simulink model "multiRobotSoccer"  (R2022b)
settings: Solver=FixedStepAuto  StartTime=0.0  StopTime=inf  FixedStep=sampleTime  RelTol=1e-3
PreLoadFcn:
  | robotSoccerParams;
values from neighbouring files (symbols this model uses):
  angThresh = pi/16    (= 0.196349540849)    [robotSoccerParams.m]
  attackerKickSpeed = 3    [robotSoccerParams.m]
  attackerMaxGoalDist = 10    [robotSoccerParams.m]
  attackerMinGoalDist = 5    [robotSoccerParams.m]
  awayGoalPosition = [fieldLimitsX(2) mean(fieldLimitsY)]    [robotSoccerParams.m]
  ballAngleNoise = pi/24    (= 0.1308996939)    [robotSoccerParams.m]
  ballThresh = robotRadius + 0.3    (= 1.1)    [robotSoccerParams.m]
  ballVelNoise = 0.5    [robotSoccerParams.m]
  defenderAwayPoses = [82 28.5 pi ... (first row only)    [robotSoccerParams.m]
  defenderHomePoses = [10 28.5 0 ... (first row only)    [robotSoccerParams.m]
  defenderKickSpeed = 5    [robotSoccerParams.m]
  distThresh = 1    [robotSoccerParams.m]
  dribbleKickSpeed = 2    [robotSoccerParams.m]
  dribbleTime = 25    [robotSoccerParams.m]
  fieldCenter = [mean(fieldLimitsX) mean(fieldLimitsY)]    [robotSoccerParams.m]
  fieldLimitsX = [0 92]    [robotSoccerParams.m]
  fieldLimitsY = [0 47]    [robotSoccerParams.m]
  goalkeeperKickSpeed = 10    [robotSoccerParams.m]
  goalkeeperPoses = [ 2 23.5 0 ... (first row only)    [robotSoccerParams.m]
  goalPosts = [ 0 33 2 ... (first row only)    [robotSoccerParams.m]
  goalThresh = 20    [robotSoccerParams.m]
  homeGoalPosition = [fieldLimitsX(1) mean(fieldLimitsY)]    [robotSoccerParams.m]
  initBallPos = fieldCenter    [robotSoccerParams.m]
  initGameState = struct('possession',0,                         'state',GameState.InPlay,                         'score',[0;0])    [robotSoccerParams.m]
  numRobots = 8    [robotSoccerParams.m]
  objColors = [0 0.75 0; 1 0 0; 0 0 1]    [robotSoccerParams.m]
  objMarkers = 'o^^'    [robotSoccerParams.m]
  outOfBoundsDist = 2    [robotSoccerParams.m]
  robotDetectorMaxHits = 5    [robotSoccerParams.m]
  robotRadius = 0.8    [robotSoccerParams.m]
undefined symbols (not defined in the file or in its folder): DiscIntNeverNeededParam, ObjectType
libraries: soccerRobotLib x8
(part 1 of 2)
settings Model: PacingRate=3  TunableVars=angThresh,attackerKickSpeed,attackerMaxGoalDist,attackerMinGoalDist,awayGoalPosition,ballAngleNoise,ballCarryFactor,ballThresh,ballVelNoise,defenderAwayPoses,defenderHomePoses,defenderKickSpeed,distThresh,dribbleKickSpeed,dribbleTime,fieldCenter,fieldLimitsX,fieldLimitsY,goalPosts,goalThresh,goalkeeperKickSpeed,goalkeeperPoses,homeGoalPosition,initBallPos,initGameState,initialPoses,numRobots,objColors,objDetectorAngle,objDetectorFOV,objDetectorMaxHits,objDetectorOffset,objDetectorRange,outOfBoundsDist,robotColors,robotDetectorAngle,robotDetectorFOV,robotDetectorMaxHits,robotDetectorOffset,robotDetectorRange,robotRadius,sampleTime,wheelRadius  TunableVarsStorageClass=Auto,Auto,Auto,Auto,Auto,Auto,Auto,Auto,Auto,Auto,Auto,Auto,Auto,Auto,Auto,Auto,Auto,Auto,Auto,Auto,Auto,Auto,Auto,Auto,Auto,Auto,Auto,Auto,Auto,Auto,Auto,Auto,Auto,Auto,Auto,Auto,Auto,Auto,Auto,Auto,Auto,Auto,Auto  TunableVarsTypeQualifier=,,,,,,,,,,,,,,,,,,,,,,,,,,,,,,,,,,,,,,,,,,  Creator=scastro  LastModifiedBy=josep
settings SolverCC: AlgebraicLoopSolver=TrustRegion
settings DataIOCC: ReturnWorkspaceOutputs=off
settings OptimizationCC: EnhancedBackFolding=on  PassReuseOutputArgsAs=Individual arguments  OptimizeBlockOrder=speed  DifferentSizesBufferReuse=on  OptimizationCustomize=off  EfficientTunableParamExpr=on
settings DebuggingCC: ParameterTunabilityLossMsg=error  UnconnectedInputMsg=warning  UnconnectedOutputMsg=warning  UnconnectedLineMsg=warning  BusObjectLabelMismatch=error  StrictBusMsg=ErrorOnBusTreatedAsVector  NonBusSignalsTreatedAsBus=error  SFMachineParentedDataDiag=warning  ArithmeticOperatorsInVariantConditions=warning
settings ModelReferenceCC: EnableRefExpFcnMdlSchedulingChecks=on
settings SFSimCC: SimUseLocalCustomCode=off  MATLABDynamicMemAlloc=off  CustomCodeUndefinedFunction=UseInterfaceOnly
settings RTWCC: Description=Embedded Coder  SystemTargetFile=ert.tlc  TemplateMakefile=ert_default_tmf  GenerateReport=on  RTWUseLocalCustomCode=off  IncludeHyperlinkInReport=on  LaunchReport=on  GenerateTraceInfo=on  GenerateTraceReport=on  GenerateTraceReportSl=on  GenerateTraceReportSf=on  GenerateTraceReportEml=on  GenerateWebview=on
settings CodeAppCC: ForceParamTrailComments=on  IgnoreCustomStorageClasses=off  OperatorAnnotations=on  SimulinkDataObjDesc=on  SFDataObjDesc=on  InsertBlockDesc=on
settings ERTTargetCC: TargetLangStandard=C99 (ISO)  GenerateSampleERTMain=on  SupportVariableSizeSignals=on  ERTCustomFileTemplate=example_file_process.tlc

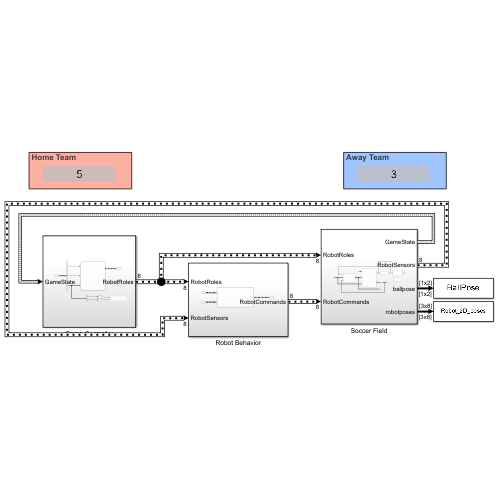
[thumbnail: Simulink's stored preview of the top-level diagram]
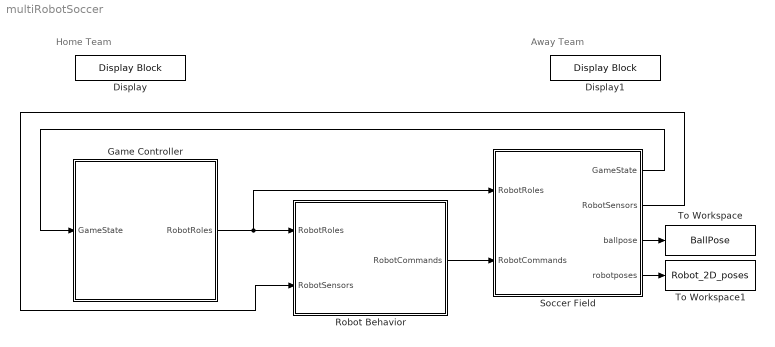
== system multiRobotSoccer ==
  note: Home Team
  note: Away Team
  Display : DisplayBlock  LabelPosition=Hide  Format=long
  Display1 : DisplayBlock  LabelPosition=Hide  Format=long
  Game Controller : Subsystem
  Robot Behavior : Subsystem
  Soccer Field : Subsystem
  To Workspace : ToWorkspace  VariableName=BallPose  SaveFormat=Structure With Time  SampleTime=-1
  To Workspace1 : ToWorkspace  VariableName=Robot_2D_poses  SaveFormat=Structure With Time  SampleTime=-1
  wires:
  Robot Behavior/1(RobotCommands) -> Soccer Field/2(RobotCommands)
  Game Controller/1(RobotRoles) -> Soccer Field/1(RobotRoles), Robot Behavior/1(RobotRoles)
  Soccer Field/1(GameState) -> Game Controller/1(GameState)
  Soccer Field/2(RobotSensors) -> Robot Behavior/2(RobotSensors)
  Soccer Field/3(ballpose) -> To Workspace/1
  Soccer Field/4(robotposes) -> To Workspace1/1

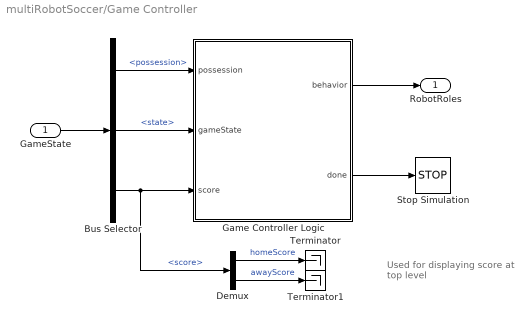
== system multiRobotSoccer/Game Controller ==
  note: Used for displaying score at top level
  GameState : Inport
  Bus Selector : BusSelector  OutputSignals=possession,state,score
  Demux : Demux  Outputs=2
  Game Controller Logic : Stateflow chart  TreatAsAtomicUnit=on
  Stop Simulation : Stop
  Terminator : Terminator
  Terminator1 : Terminator
  RobotRoles : Outport  VectorParamsAs1DForOutWhenUnconnected=off
  wires:
  Game Controller Logic/1(behavior) -> RobotRoles/1
  GameState/1 -> Bus Selector/1
  Bus Selector/1 -> Game Controller Logic/1(possession)  "<possession>"
  Bus Selector/2 -> Game Controller Logic/2(gameState)  "<state>"
  Bus Selector/3 -> Demux/1, Game Controller Logic/3(score)  "<score>"
  Demux/1 -> Terminator/1  "homeScore"
  Demux/2 -> Terminator1/1  "awayScore"
  Game Controller Logic/2(done) -> Stop Simulation/1

== system multiRobotSoccer/Robot Behavior ==
  RobotRoles : Inport
  RobotSensors : Inport  Port=2
  For Each Subsystem (Iterates through all robots) : Subsystem  TreatAsAtomicUnit=on
  RobotCommands : Outport  OutDataTypeStr=Bus: RobotCommandBus  PortDimensions=2  VectorParamsAs1DForOutWhenUnconnected=off
  wires:
  RobotRoles/1 -> For Each Subsystem (Iterates through all robots)/1(robotRoles)
  RobotSensors/1 -> For Each Subsystem (Iterates through all robots)/2(robotSensors)
  For Each Subsystem (Iterates through all robots)/1(robotCommands) -> RobotCommands/1

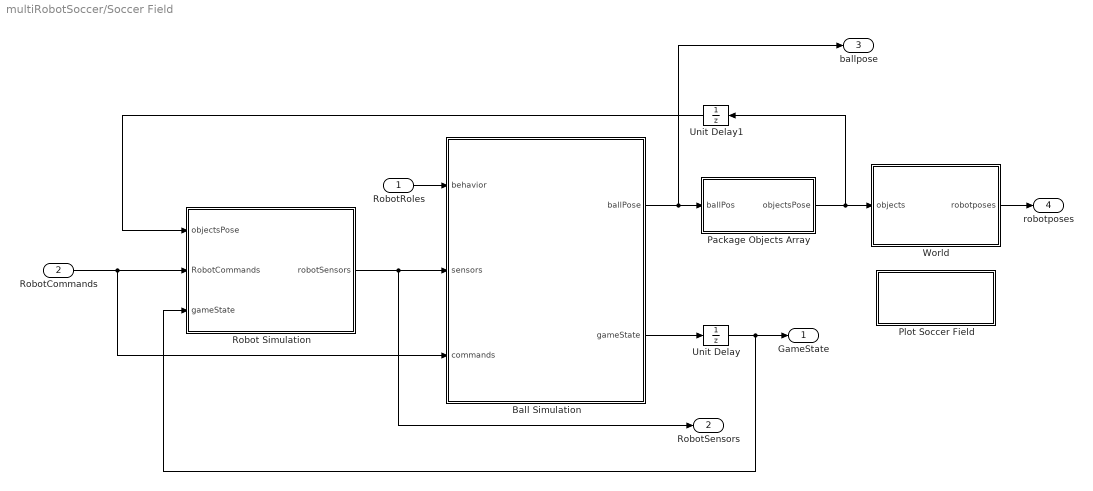
== system multiRobotSoccer/Soccer Field ==
  RobotRoles : Inport
  RobotCommands : Inport  Port=2
  Ball Simulation : Stateflow chart  TreatAsAtomicUnit=on
  Package Objects Array : Subsystem
  Plot Soccer Field : MATLAB Function  TreatAsAtomicUnit=on
  Robot Simulation : Subsystem
  Unit Delay : UnitDelay  InitialCondition=initGameState  SampleTime=-1  HasFrameUpgradeWarning=on
  Unit Delay1 : UnitDelay  InitialCondition=[initBallPos double(ObjectType.Ball); goalPosts]  SampleTime=-1  HasFrameUpgradeWarning=on
  World : Subsystem  AncestorBlock=mobileRoboticsLib/Environments/Multi-Robot Environment  InitFcn=clear multiRobotVizWorld;  mask(Multi-Robot Environment){numRobots=numRobots, mapName=map, showWaypoints=off, showObjects=on, objectColors=objColors, objectMarkers=objMarkers, showRobotIds=off, plotSensorLines=off}
      mask prompts: numRobots "Number of Robots"; mapName "Map Name"; showWaypoints "Accept Waypoints"; showObjects "Accept Objects"; objectColors "Object Colors"; objectMarkers "Object Markers"; showRobotIds "Show Robot IDs"; plotSensorLines "Plot Sensor Lines"
      mask help:
      | Displays map, waypoint, and object data for a multi-robot simulation.
      |
      | Use "Multi-Robot Visualizer" blocks to display individual robots in this environment.
      mask init:
      | % Configure visual tags
      | visualSub = [gcb '/Visuals'];
      | radiusBlocks = find_system(visualSub,'FollowLinks','on','LookUnderMasks','on','BlockType','From');
      | for idx = 1:numel(radiusBlocks)
      |     lh = get_param(radiusBlocks{idx},'LineHandles');
      |     delete_line(lh.Outport);
      | end
      | delete_block(radiusBlocks);
      | vecBlock = [visualSub '/Vector Concatenate'];
      | set_param(vecBlock,'NumInputs',num2str(numRobots));
      | for idx = 1:numRobots
      |     blkName = [visualSub '/From' num2str(idx)];
      |     blkPos = [0 30 200 50] + (idx-1)*[0 30 0 30];
      |     add_block('simulink/Signal Routing/From',blkName);
      |     set_param(blkName,'GotoTag',['slMultiRobotEnv_Visuals_' num2str(idx)]);
      |     set_param(blkName,'Position',blkPos);
      |     add_line(visualSub,['From' num2str(idx) '/1'],['Vector Concatenate/' num2str(idx)]);
      | end
      | 
      | % Configure pose tags
      | poseSub = [gcb '/Poses'];
      | poseBlocks = find_system(poseSub,'FollowLinks','on','LookUnderMasks','on','BlockType','From');
      | for idx = 1:numel(poseBlocks)
      |     lh = get_param(poseBlocks{idx},'LineHandles');
      |     delete_line(lh.Outport);
      | end
      | delete_block(poseBlocks);
      | vecBlock = [poseSub '/Vector Concatenate'];
      | set_param(vecBlock,'NumInputs',num2str(numRobots));
      | for idx = 1:numRobots
      |     blkName = [poseSub '/From' num2str(idx)];
      |     blkPos = [0 30 200 50] + (idx-1)*[0 30 0 30];
      |     add_block('simulink/Signal Routing/From',blkName);
      |     set_param(blkName,'GotoTag',['slMultiRobotEnv_Pose_' num2str(idx)]);
      |     set_param(blkName,'Position',blkPos);
      |     add_line(poseSub,['From' num2str(idx) '/1'],['Vector Concatenate/' num2str(idx)]);
      | end
      | 
      | % Configure range tags
      | rangeSub = [gcb '/Ranges'];
      | rangeBlocks = find_system(rangeSub,'FollowLinks','on','LookUnderMasks','on','BlockType','From');
      | for idx = 1:numel(rangeBlocks)
      |     lh = get_param(rangeBlocks{idx},'LineHandles');
      |     delete_line(lh.Outport);
      | end
      | delete_block(rangeBlocks);
      | vecBlock = [rangeSub '/Vector Concatenate'];
      | set_param(vecBlock,'NumInputs',num2str(numRobots));
      | for idx = 1:numRobots
      |     blkName = [rangeSub '/From' num2str(idx)];
      |     blkPos = [0 30 200 50] + (idx-1)*[0 30 0 30];
      |     add_block('simulink/Signal Routing/From',blkName);
      |     set_param(blkName,'GotoTag',['slMultiRobotEnv_Ranges_' num2str(idx)]);
      |     set_param(blkName,'Position',blkPos);
      |     add_line(rangeSub,['From' num2str(idx) '/1'],['Vector Concatenate/' num2str(idx)]);
      | end
      | 
      | % Initialize range sensor bus
      | internal.createRangeSensorBus;
      | 
      | % Configure object detector tags
      | objDetSub = [gcb '/ObjectDetectorParams'];
      | objDetBlocks = find_system(objDetSub,'FollowLinks','on','LookUnderMasks','on','BlockType','From');
      | for idx = 1:numel(objDetBlocks)
      |     lh = get_param(objDetBlocks{idx},'LineHandles');
      |     delete_line(lh.Outport);
      | end
      | delete_block(objDetBlocks);
      | vecBlock = [objDetSub '/Vector Concatenate'];
      | set_param(vecBlock,'NumInputs',num2str(numRobots));
      | for idx = 1:numRobots
      |     blkName = [objDetSub '/From' num2str(idx)];
      |     blkPos = [0 30 200 50] + (idx-1)*[0 30 0 30];
      |     add_block('simulink/Signal Routing/From',blkName);
      |     set_param(blkName,'GotoTag',['slMultiRobotEnv_ObjDet_' num2str(idx)]);
      |     set_param(blkName,'Position',blkPos);
      |     add_line(objDetSub,['From' num2str(idx) '/1'],['Vector Concatenate/' num2str(idx)]);
      | end
      | 
      | % Configure robot detector tags
      | robotDetSub = [gcb '/RobotDetectorParams'];
      | robotDetBlocks = find_system(robotDetSub,'FollowLinks','on','LookUnderMasks','on','BlockType','From');
      | for idx = 1:numel(robotDetBlocks)
      |     lh = get_param(robotDetBlocks{idx},'LineHandles');
      |     delete_line(lh.Outport);
      | end
      | delete_block(robotDetBlocks);
      | vecBlock = [robotDetSub '/Vector Concatenate'];
      | set_param(vecBlock,'NumInputs',num2str(numRobots));
      | for idx = 1:numRobots
      |     blkName = [robotDetSub '/From' num2str(idx)];
      |     blkPos = [0 30 200 50] + (idx-1)*[0 30 0 30];
      |     add_block('simulink/Signal Routing/From',blkName);
      |     set_param(blkName,'GotoTag',['slMultiRobotEnv_RobotDet_' num2str(idx)]);
      |     set_param(blkName,'Position',blkPos);
      |     add_line(robotDetSub,['From' num2str(idx) '/1'],['Vector Concatenate/' num2str(idx)]);
      | end
      | 
      | % Configure waypoints port
      | hasWaypointPort = ~isempty(find_system(gcb,'FollowLinks','on','LookUnderMasks','on','BlockType','Inport','Name','waypoints'));
      | if ~showWaypoints & hasWaypointPort
      |     replace_block(gcb,'FollowLinks','on','Name','waypoints','built-in/Ground','noprompt');
      | elseif showWaypoints & ~hasWaypointPort
      |     replace_block(gcb,'FollowLinks','on','Name','waypoints','built-in/Inport','noprompt'); 
      | end
      |  
      | % Configure objects port
      | hasObjectPort = ~isempty(find_system(gcb,'FollowLinks','on','LookUnderMasks','on','BlockType','Inport','Name','objects'));
      | if ~showObjects & hasObjectPort
      |     replace_block(gcb,'FollowLinks','on','Name','objects','built-in/Ground','noprompt');
      | elseif showObjects & ~hasObjectPort
      |     replace_block(gcb,'FollowLinks','on','Name','objects','built-in/Inport','noprompt');  
      | end
      | 
      | % Ensure the waypoints and objects ports are organized correctly
      | if strcmp(get_param([gcb '/waypoints'],'BlockType'),'Inport')
      |     set_param([gcb '/waypoints'],'Port','1');
      | end
      settings: LibrarySourceBlock=mobileRoboticsLib/Environments/Multi-Robot Environment
      mask Help: web('matlab: edit mrsDocMultiRobotEnv')
      mask Callback showObjects:
      | mask = Simulink.Mask.get(gcb);
      | showObjects = get_param(gcb,'showObjects');
      | 
      | % Enable and disable parameters
      | indices = [find(strcmp({mask.Parameters.Name},'objectColors'));
      |            find(strcmp({mask.Parameters.Name},'objectMarkers'))];
      | 
      | for idx = 1:numel(indices)
      |     mask.Parameters(indices(idx)).Visible = showObjects;
      | end
      mask Display: fprintf('Multi-Robot\nEnvironment')
  GameState : Outport  VectorParamsAs1DForOutWhenUnconnected=off
  RobotSensors : Outport  Port=2  VectorParamsAs1DForOutWhenUnconnected=off
  ballpose : Outport  Port=3
  robotposes : Outport  Port=4
  wires:
  Package Objects Array/1(objectsPose) -> World/1(objects), Unit Delay1/1
  Ball Simulation/1(ballPose) -> ballpose/1, Package Objects Array/1(ballPos)
  RobotCommands/1 -> Robot Simulation/2(RobotCommands), Ball Simulation/3(commands)
  Ball Simulation/2(gameState) -> Unit Delay/1
  Unit Delay1/1 -> Robot Simulation/1(objectsPose)
  Unit Delay/1 -> Robot Simulation/3(gameState), GameState/1
  Robot Simulation/1(robotSensors) -> RobotSensors/1, Ball Simulation/2(sensors)
  RobotRoles/1 -> Ball Simulation/1(behavior)
  World/1(robotposes) -> robotposes/1

== system multiRobotSoccer/Robot Behavior/For Each Subsystem (Iterates through all robots) ==
  robotRoles : Inport  Partition=on  PartitionDimension=1  PartitionWidth=1  PartitionOffset=0
  robotSensors : Inport  Port=2  Partition=on  PartitionDimension=1  PartitionWidth=1  PartitionOffset=0
  For Each : ForEach  DisableCoverage=on
  SoccerBehavior : Stateflow chart  TreatAsAtomicUnit=on
  robotCommands : Outport  ConcatenationDimension=1  VectorParamsAs1DForOutWhenUnconnected=off
  wires:
  SoccerBehavior/1(commands) -> robotCommands/1
  robotRoles/1 -> SoccerBehavior/2(behavior)
  robotSensors/1 -> SoccerBehavior/1(sensors)

== system multiRobotSoccer/Soccer Field/Ball Simulation/BallDynamics.InBounds.BallFree ==
  Action Port : ActionPort
      settings: CopyFcn=Stateflow.SLINSF.SimulinkMan.removeBlockPreDeleteFcn  PreDeleteFcn=Stateflow.SLINSF.SimulinkMan.unsafePredeleteFcn
  Gain : Gain  Gain=-0.25
  Position Integrator : DiscreteIntegrator  InitialCondition=initBallPos  SampleTime=-1  StateName=ballPos  ICPrevOutput=DiscIntNeverNeededParam  ICPrevScaledInput=DiscIntNeverNeededParam
  Signal Specification : SignalSpecification  Dimensions=[1 2]
  Velocity Integrator : DiscreteIntegrator  InitialCondition=[0 0]  SampleTime=-1  StateName=ballVel  ICPrevOutput=DiscIntNeverNeededParam  ICPrevScaledInput=DiscIntNeverNeededParam
  ballPose : Outport  VectorParamsAs1DForOutWhenUnconnected=off
  wires:
  Gain/1 -> Velocity Integrator/1
  Velocity Integrator/1 -> Signal Specification/1
  Position Integrator/1 -> ballPose/1
  Signal Specification/1 -> Position Integrator/1, Gain/1

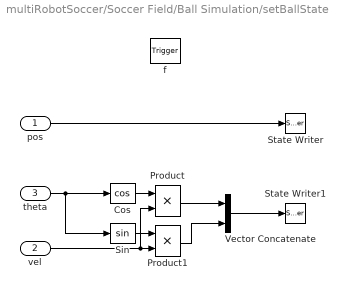
== system multiRobotSoccer/Soccer Field/Ball Simulation/setBallState ==
  pos : Inport  OutDataTypeStr=double  PortDimensions=[1 2]
  vel : Inport  Port=2  OutDataTypeStr=double  PortDimensions=1
  theta : Inport  Port=3  OutDataTypeStr=double  PortDimensions=1
  f : TriggerPort  TriggerType=function-call  VariantControl=(inherit)
      settings: CopyFcn=Stateflow.SLINSF.SimulinkMan.removeBlockPreDeleteFcn  PreDeleteFcn=Stateflow.SLINSF.SimulinkMan.unsafePredeleteFcn
  Cos : Trigonometry  Operator=cos
  Product : Product
  Product1 : Product
  Sin : Trigonometry
  State Writer : StateWriter  StateOwnerBlock=../../BallDynamics.InBounds.BallFree/Position Integrator  StateName=ballPos
  State Writer1 : StateWriter  StateOwnerBlock=../../BallDynamics.InBounds.BallFree/Velocity Integrator  StateName=ballVel
  Vector Concatenate : Concatenate  Mode=Multidimensional array  ConcatenateDimension=2
  wires:
  Vector Concatenate/1 -> State Writer1/1
  Product1/1 -> Vector Concatenate/2
  Product/1 -> Vector Concatenate/1
  theta/1 -> Cos/1, Sin/1
  Sin/1 -> Product1/1
  vel/1 -> Product1/2, Product/2
  Cos/1 -> Product/1
  pos/1 -> State Writer/1

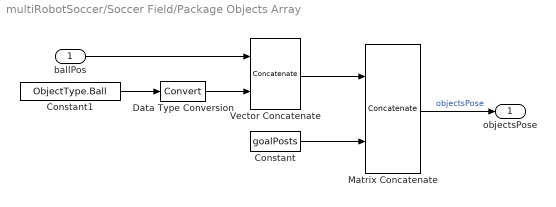
== system multiRobotSoccer/Soccer Field/Package Objects Array ==
  ballPos : Inport
  Constant : Constant  Value=goalPosts  VectorParams1D=off
  Constant1 : Constant  Value=ObjectType.Ball
  Data Type Conversion : DataTypeConversion  SaturateOnIntegerOverflow=off  RndMeth=Floor
  Matrix Concatenate : Concatenate  Mode=Multidimensional array
  Vector Concatenate : Concatenate  Mode=Multidimensional array  ConcatenateDimension=2
  objectsPose : Outport  VectorParamsAs1DForOutWhenUnconnected=off
  wires:
  Constant/1 -> Matrix Concatenate/2
  Matrix Concatenate/1 -> objectsPose/1  "objectsPose"
  Vector Concatenate/1 -> Matrix Concatenate/1
  ballPos/1 -> Vector Concatenate/1
  Constant1/1 -> Data Type Conversion/1
  Data Type Conversion/1 -> Vector Concatenate/2

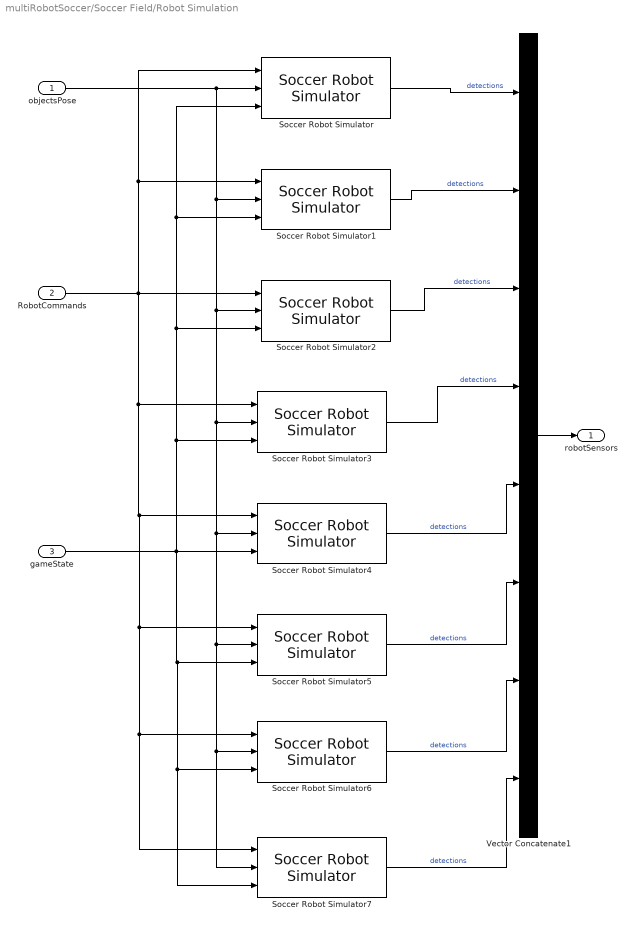
== system multiRobotSoccer/Soccer Field/Robot Simulation ==
  objectsPose : Inport
  RobotCommands : Inport  Port=2
  gameState : Inport  Port=3
  Soccer Robot Simulator : soccerRobotLib/Soccer Robot Simulator  robotIdx=1
  Soccer Robot Simulator1 : soccerRobotLib/Soccer Robot Simulator  robotIdx=2
  Soccer Robot Simulator2 : soccerRobotLib/Soccer Robot Simulator  robotIdx=3
  Soccer Robot Simulator3 : soccerRobotLib/Soccer Robot Simulator  robotIdx=4
  Soccer Robot Simulator4 : soccerRobotLib/Soccer Robot Simulator  robotIdx=5
  Soccer Robot Simulator5 : soccerRobotLib/Soccer Robot Simulator  robotIdx=6
  Soccer Robot Simulator6 : soccerRobotLib/Soccer Robot Simulator  robotIdx=7
      link override Visualize Robot 1/Goto_ObjDetector: GotoTag=slMultiRobotEnv_Visuals_7
      link override Visualize Robot 1/Goto_Pose: GotoTag=slMultiRobotEnv_Visuals_7
      link override Visualize Robot 1/Goto_Ranges: GotoTag=slMultiRobotEnv_Visuals_7
      link override Visualize Robot 1/Goto_RobotDetector: GotoTag=slMultiRobotEnv_Visuals_7
      link override Visualize Robot 1/Goto_Visuals: GotoTag=slMultiRobotEnv_Visuals_7
  Soccer Robot Simulator7 : soccerRobotLib/Soccer Robot Simulator  robotIdx=8
      link override Visualize Robot 1/Goto_ObjDetector: GotoTag=slMultiRobotEnv_Pose_8
      link override Visualize Robot 1/Goto_Pose: GotoTag=slMultiRobotEnv_Pose_8
      link override Visualize Robot 1/Goto_Ranges: GotoTag=slMultiRobotEnv_Pose_8
      link override Visualize Robot 1/Goto_RobotDetector: GotoTag=slMultiRobotEnv_Pose_8
      link override Visualize Robot 1/Goto_Visuals: GotoTag=slMultiRobotEnv_Visuals_8
  Vector Concatenate1 : Concatenate  NumInputs=8
  robotSensors : Outport  VectorParamsAs1DForOutWhenUnconnected=off
  wires:
  RobotCommands/1 -> Soccer Robot Simulator/1, Soccer Robot Simulator1/1, Soccer Robot Simulator3/1, Soccer Robot Simulator7/1, Soccer Robot Simulator6/1, Soccer Robot Simulator5/1, Soccer Robot Simulator4/1, Soccer Robot Simulator2/1
  objectsPose/1 -> Soccer Robot Simulator/2, Soccer Robot Simulator1/2, Soccer Robot Simulator7/2, Soccer Robot Simulator6/2, Soccer Robot Simulator5/2, Soccer Robot Simulator4/2, Soccer Robot Simulator3/2, Soccer Robot Simulator2/2
  Vector Concatenate1/1 -> robotSensors/1
  Soccer Robot Simulator/1 -> Vector Concatenate1/1  "detections"
  Soccer Robot Simulator1/1 -> Vector Concatenate1/2  "detections"
  Soccer Robot Simulator2/1 -> Vector Concatenate1/3  "detections"
  Soccer Robot Simulator3/1 -> Vector Concatenate1/4  "detections"
  gameState/1 -> Soccer Robot Simulator7/3, Soccer Robot Simulator6/3, Soccer Robot Simulator5/3, Soccer Robot Simulator/3, Soccer Robot Simulator1/3, Soccer Robot Simulator2/3, Soccer Robot Simulator3/3, Soccer Robot Simulator4/3
  Soccer Robot Simulator4/1 -> Vector Concatenate1/5  "detections"
  Soccer Robot Simulator5/1 -> Vector Concatenate1/6  "detections"
  Soccer Robot Simulator6/1 -> Vector Concatenate1/7  "detections"
  Soccer Robot Simulator7/1 -> Vector Concatenate1/8  "detections"

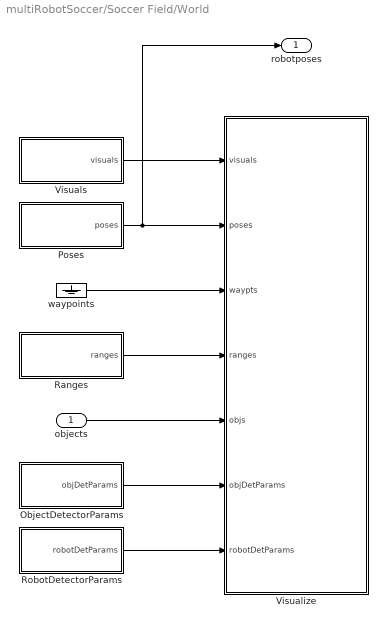
== system multiRobotSoccer/Soccer Field/World ==
  objects : Inport
  ObjectDetectorParams : Subsystem
  Poses : Subsystem
  Ranges : Subsystem
  RobotDetectorParams : Subsystem
  Visualize : MATLAB Function  TreatAsAtomicUnit=on
  Visuals : Subsystem
  waypoints : Ground
  robotposes : Outport
  wires:
  objects/1 -> Visualize/5(objs)
  waypoints/1 -> Visualize/3(waypts)
  Ranges/1(ranges) -> Visualize/4(ranges)
  Poses/1(poses) -> robotposes/1, Visualize/2(poses)
  Visuals/1(visuals) -> Visualize/1(visuals)
  ObjectDetectorParams/1(objDetParams) -> Visualize/6(objDetParams)
  RobotDetectorParams/1(robotDetParams) -> Visualize/7(robotDetParams)

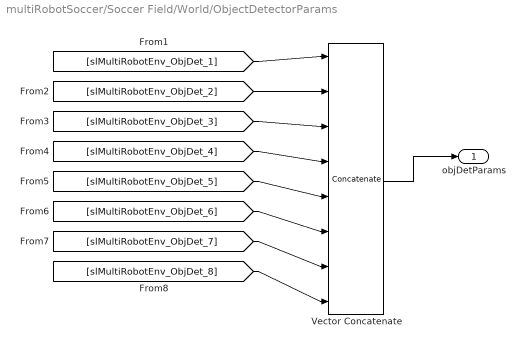
== system multiRobotSoccer/Soccer Field/World/ObjectDetectorParams ==
  Vector Concatenate : Concatenate  NumInputs=8  Mode=Multidimensional array  ConcatenateDimension=2
  objDetParams : Outport
  wires:
  Vector Concatenate/1 -> objDetParams/1
  [slMultiRobotEnv_ObjDet_1] -> Vector Concatenate/1
  [slMultiRobotEnv_ObjDet_2] -> Vector Concatenate/2
  [slMultiRobotEnv_ObjDet_3] -> Vector Concatenate/3
  [slMultiRobotEnv_ObjDet_4] -> Vector Concatenate/4
  [slMultiRobotEnv_ObjDet_5] -> Vector Concatenate/5
  [slMultiRobotEnv_ObjDet_6] -> Vector Concatenate/6
  [slMultiRobotEnv_ObjDet_7] -> Vector Concatenate/7
  [slMultiRobotEnv_ObjDet_8] -> Vector Concatenate/8

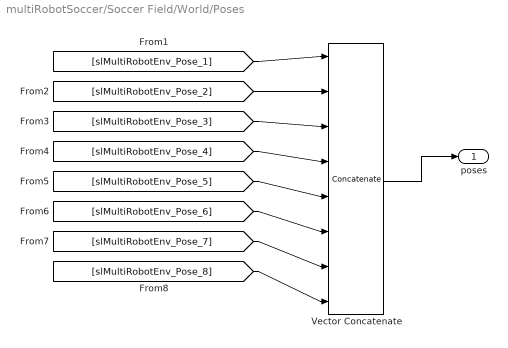
== system multiRobotSoccer/Soccer Field/World/Poses ==
  Vector Concatenate : Concatenate  NumInputs=8  Mode=Multidimensional array  ConcatenateDimension=2
  poses : Outport
  wires:
  Vector Concatenate/1 -> poses/1
  [slMultiRobotEnv_Pose_1] -> Vector Concatenate/1
  [slMultiRobotEnv_Pose_2] -> Vector Concatenate/2
  [slMultiRobotEnv_Pose_3] -> Vector Concatenate/3
  [slMultiRobotEnv_Pose_4] -> Vector Concatenate/4
  [slMultiRobotEnv_Pose_5] -> Vector Concatenate/5
  [slMultiRobotEnv_Pose_6] -> Vector Concatenate/6
  [slMultiRobotEnv_Pose_7] -> Vector Concatenate/7
  [slMultiRobotEnv_Pose_8] -> Vector Concatenate/8

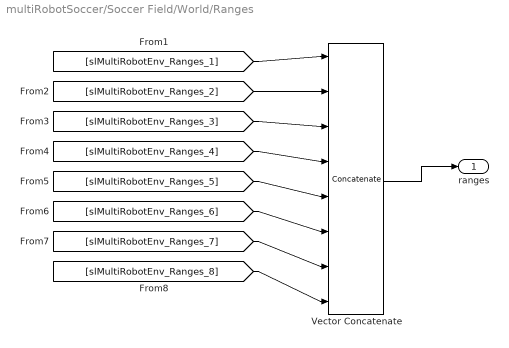
== system multiRobotSoccer/Soccer Field/World/Ranges ==
  Vector Concatenate : Concatenate  NumInputs=8  Mode=Multidimensional array  ConcatenateDimension=2
  ranges : Outport
  wires:
  Vector Concatenate/1 -> ranges/1
  [slMultiRobotEnv_Ranges_1] -> Vector Concatenate/1
  [slMultiRobotEnv_Ranges_2] -> Vector Concatenate/2
  [slMultiRobotEnv_Ranges_3] -> Vector Concatenate/3
  [slMultiRobotEnv_Ranges_4] -> Vector Concatenate/4
  [slMultiRobotEnv_Ranges_5] -> Vector Concatenate/5
  [slMultiRobotEnv_Ranges_6] -> Vector Concatenate/6
  [slMultiRobotEnv_Ranges_7] -> Vector Concatenate/7
  [slMultiRobotEnv_Ranges_8] -> Vector Concatenate/8

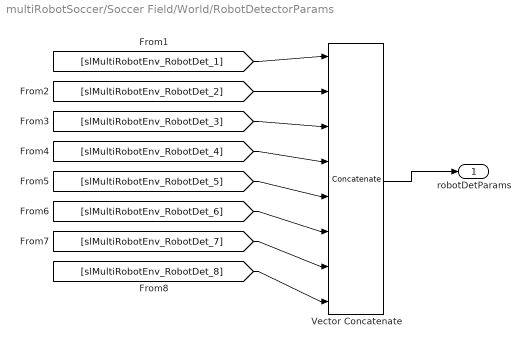
== system multiRobotSoccer/Soccer Field/World/RobotDetectorParams ==
  Vector Concatenate : Concatenate  NumInputs=8  Mode=Multidimensional array  ConcatenateDimension=2
  robotDetParams : Outport
  wires:
  Vector Concatenate/1 -> robotDetParams/1
  [slMultiRobotEnv_RobotDet_1] -> Vector Concatenate/1
  [slMultiRobotEnv_RobotDet_2] -> Vector Concatenate/2
  [slMultiRobotEnv_RobotDet_3] -> Vector Concatenate/3
  [slMultiRobotEnv_RobotDet_4] -> Vector Concatenate/4
  [slMultiRobotEnv_RobotDet_5] -> Vector Concatenate/5
  [slMultiRobotEnv_RobotDet_6] -> Vector Concatenate/6
  [slMultiRobotEnv_RobotDet_7] -> Vector Concatenate/7
  [slMultiRobotEnv_RobotDet_8] -> Vector Concatenate/8

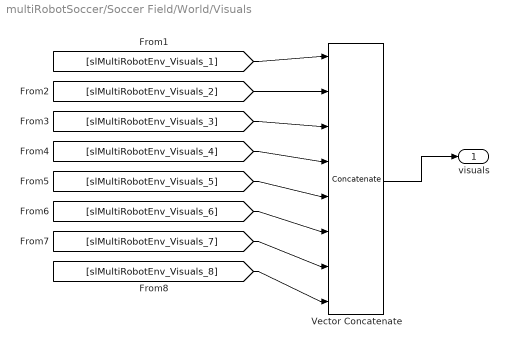
== system multiRobotSoccer/Soccer Field/World/Visuals ==
  Vector Concatenate : Concatenate  NumInputs=8  Mode=Multidimensional array  ConcatenateDimension=2
  visuals : Outport
  wires:
  Vector Concatenate/1 -> visuals/1
  [slMultiRobotEnv_Visuals_1] -> Vector Concatenate/1
  [slMultiRobotEnv_Visuals_2] -> Vector Concatenate/2
  [slMultiRobotEnv_Visuals_3] -> Vector Concatenate/3
  [slMultiRobotEnv_Visuals_4] -> Vector Concatenate/4
  [slMultiRobotEnv_Visuals_5] -> Vector Concatenate/5
  [slMultiRobotEnv_Visuals_6] -> Vector Concatenate/6
  [slMultiRobotEnv_Visuals_7] -> Vector Concatenate/7
  [slMultiRobotEnv_Visuals_8] -> Vector Concatenate/8

== stateflow chart multiRobotSoccer/Soccer Field/Ball Simulation ==
  state BallPossession [parallel]
    en:
    gameState.possession = 0;
    en,du:
    % Calculate distances from robots to ball
    % (Goalkeepers get 2x the range)
    for idx = 1:numRobots
    ballDists(idx) = norm( sensors(idx).pose(1:2) - ballPose' );
    if behavior(idx).role == Role.Goalkeeper
    ballDists(idx) = ballDists(idx)/2;
    end
    end
    % Find the robot index of the current and latest possessions
    robotIdx = findPossession;
    if robotIdx > 0
    lastPossession = robotIdx;
    end
    % Unpack the robot commands
    action = commands(lastPossession).action;
    ballVel = commands(lastPossession).ballVelocity;
    robotPose = sensors(lastPossession).pose;
    settings: executionOrder=1
  state BallDynamics [parallel]
    en:
    coder.extrinsic('randn'); % Lets us use MATLAB's interpreted RNG
    setBallState(initBallPos,0,0);
    settings: executionOrder=2
    state InBounds
      en, du:
      randNum = randn(2,1);
      gameState.state = getGameState;
      state BallFree
      state BallHeld
        en: gameState.possession = robotIdx;
        en,du:
        ballPose = [robotPose(1) robotPose(2)] + ...
        (robotRadius+ballThresh)*[cos(robotPose(3)) sin(robotPose(3))];
      (default) -> BallFree
      BallHeld -> BallFree : [action == RobotAction.KickBall]
          | {setBallState(ballPose,ballVel + ballVelNoise*randNum(1), ...
          |  robotPose(3) + ballAngleNoise*randNum(2));
          | gameState.possession = 0;}
      BallFree -> BallHeld : [after(2,sec) && ...
          |  robotIdx > 0]
    state OutOfBounds
      en:
      % If a goal is scored, increment the score
      if gameState.state == GameState.GoalScored
      ballPose = initBallPos;
      teamIdx = behavior(lastPossession).team;
      gameState.score(teamIdx) = gameState.score(teamIdx) + 1;
      % Else, place the ball back in bounds
      else
      ballPose = placeBallInBounds();
      end
      setBallState(ballPose,0,robotPose(3));
    (default) -> InBounds
    OutOfBounds -> InBounds : after(1,sec)
    InBounds -> OutOfBounds : [gameState.state ~= GameState.InPlay]
  state setBallState(pos,vel,theta) [function]
  state rIdx = findPossession [function]
    (default) -> (junction 125)
    (junction 125) -> (junction 127) [order 1] : % If the robot that previously possessed the ball is still holding it, keep the same index
        | [(gameState.possession > 0) && ...
        | (commands(gameState.possession).action == RobotAction.HoldBall)]
    (junction 125) -> (junction 131) [order 2] : % Else, find another valid robot holder
        | {rIdx = findNearestHoldingRobot;}
    (junction 127) -> (junction 129) : {rIdx = gameState.possession;}
    (junction 129) -> (junction 131)
  state state = getGameState [function]
    note: Returns the game state depending on the position of the ball on the field
    (default) -> (junction 98)
    (junction 98) -> (junction 100) [order 1] : [ballPose(1) <= fieldLimitsX(1) || ballPose(1) >= fieldLimitsX(2) || ...
        |  ballPose(2) <= fieldLimitsY(1) || ballPose(2) >= fieldLimitsY(2)]
    (junction 98) -> (junction 111) [order 2] : {state = GameState.InPlay;}
    (junction 100) -> (junction 102)
    (junction 102) -> (junction 104) [order 1] : [ballPose(2)<=goalPosts(1,2) && ...
        | ballPose(2) >= goalPosts(2,2)]
    (junction 102) -> (junction 108) [order 2] : {state = GameState.OutOfPlay;}
    (junction 104) -> (junction 106) : {state = GameState.GoalScored;}
    (junction 108) -> (junction 111)
    (junction 106) -> (junction 108)
  state newPose = placeBallInBounds [function]
    note: Calculates the new pose of the ball when returning from out of bounds
    (default) -> (junction 90) : {
        | newPose = [ ...
        |  max( fieldLimitsX(1)+outOfBoundsDist , min(ballPose(1),fieldLimitsX(2)-outOfBoundsDist) ), ...
        | max( fieldLimitsY(1)+outOfBoundsDist , min(ballPose(2),fieldLimitsY(2)-outOfBoundsDist) ) ...
        | ];
        | }
  data: sf_internal_action_state_placeholder_data local double size=1 =0; pos function_input double size=[1 2]; vel function_input double size=1; theta function_input double size=1; nearIdx function_output size=1; rIdx function_output; state function_output; newPose function_output; behavior input Bus: RobotBehaviorBus; sensors input Bus: RobotSensorBus size=numRobots; ballPose output; commands input Bus: RobotCommandBus size=numRobots; robotRadius parameter; robotPose local =[0 0 0]'; action local =RobotAction.DoNothing; gameState output Bus: GameStateBus size=1; robotIdx local =1; lastPossession local =1; initBallPos parameter; randNum local =[0;0]; teamIdx local =1; ballVel local =0; ballThresh parameter; numRobots parameter; idx local =0; ballVelNoise parameter; ballAngleNoise parameter; outOfBoundsDist parameter; fieldLimitsY parameter; fieldLimitsX parameter; ballDists local =zeros(numRobots,1); goalPosts parameter
  function nearIdx = findNearestHoldingRobot:
    | function rIdx = findNearestHoldingRobot
    | % Finds possession based on the commands to all the robots 
    | % and their distances to the ball
    | 
    | [~,inds] = sort(ballDists);
    | rIdx = 0;
    | for idx = 1:numRobots
    |     if (commands(inds(idx)).action == RobotAction.HoldBall) && ....
    |        (ballDists(inds(idx)) <= ballThresh)
    |         rIdx = inds(idx);
    |         return;
    |     end
    | end
    | 
    | end

== matlab function multiRobotSoccer/Soccer Field/Plot Soccer Field ==
function plotSoccerField
% Plots the soccer field once the figure window for the environment has
% been initialized

coder.extrinsic('evalin');
persistent hasPlotted
if isempty(hasPlotted)
    evalin('base','plotSoccerField');
    hasPlotted = true;
end

== stateflow chart multiRobotSoccer/Game Controller/Game Controller Logic ==
  state GameOn
    en:
    done = false;
    % Assign player strategy
    assignRobotStrategies
    % Constantly check possession
    en,du:
    if possession > 0
    posTeam = behavior(possession).team;
    else
    posTeam = 0;
    end
    for idx = 1:numRobots
    behavior(idx).possessingTeam = posTeam;
    end
    state HomeTeamAttacks
      en:
      behavior(1).role = Role.Goalkeeper;
      behavior(2).role = Role.Goalkeeper;
      behavior(3).role = Role.Attacker;
      behavior(4).role = Role.Attacker;
      behavior(5).role = Role.Defender;
      behavior(6).role = Role.Defender;
      behavior(7).role = Role.Defender;
      behavior(8).role = Role.Defender;
    state HomeTeamDefends
      en:
      behavior(1).role = Role.Goalkeeper;
      behavior(2).role = Role.Goalkeeper;
      behavior(3).role = Role.Attacker;
      behavior(4).role = Role.Attacker;
      behavior(5).role = Role.Defender;
      behavior(6).role = Role.Defender;
      behavior(7).role = Role.Defender;
      behavior(8).role = Role.Defender;
    (default) -> HomeTeamAttacks
    HomeTeamAttacks -> HomeTeamDefends : [hasChangedFrom(gameState,GameState.InPlay) || ...
        |  posTeam == 2]
    HomeTeamDefends -> HomeTeamAttacks : [hasChangedFrom(gameState,GameState.InPlay) || ...
        |  posTeam == 1]
  state assignRobotStrategies [function]
    note: Assigns initial robot teams, roles, and default formation poses
    (default) -> (junction 54) : {
        | % Assign teams
        | behavior(1).team = 1;
        | behavior(2).team = 2;
        | behavior(3).team = 1;
        | behavior(4).team = 2;
        | behavior(5).team = 1;
        | behavior(6).team = 2;
        | behavior(7).team = 1;
        | behavior(8).team = 2;
        | }
    (junction 54) -> (junction 56) : {
        | % Assign goalkeeper roles and default poses
        | behavior(1).role = Role.Goalkeeper;
        | behavior(1).formationPose = goalkeeperPoses(:,1);
        | behavior(2).role = Role.Goalkeeper;
        | behavior(2).formationPose = goalkeeperPoses(:,2);
        | }
    (junction 56) -> (junction 58) : {
        | % Assign defender default poses
        | behavior(3).formationPose = defenderHomePoses(:,1);
        | behavior(4).formationPose = defenderAwayPoses(:,1);
        | behavior(5).formationPose = defenderHomePoses(:,2);
        | behavior(6).formationPose = defenderAwayPoses(:,2);
        | behavior(7).formationPose = defenderHomePoses(:,3);
        | behavior(8).formationPose = defenderAwayPoses(:,3);
        | }
  state GameOver
    en:
    done = true;
  (default) -> GameOn
  GameOn -> GameOver : % End the game when a team scores 5
      | [any(score >= 5)]
  data: possession input; gameState input; score input; behavior output Bus: RobotBehaviorBus size=numRobots; numRobots local =numRobots; idx local =1; posTeam local size=1 =0; defenderAwayPoses parameter; defenderHomePoses parameter; goalkeeperPoses parameter; done output
